simulink model "chap7_8sim"  (Simulink 10.3)
settings: Solver=ode45  StartTime=0.0  StopTime=6  RelTol=1e-3  EnableMultiTasking=on
settings Model: Creator=shipe  LastModifiedBy=shipe
settings SolverCC: AlgebraicLoopSolver=Auto
settings DataIOCC: LimitDataPoints=on  SignalLoggingName=sigsOut
settings OptimizationCC: ExpressionDepthLimit=128  LifeSpan=auto
settings DebuggingCC: SaveWithParameterizedLinksMsg=none  SignalResolutionControl=TryResolveAllWithWarning  MultiTaskDSMMsg=warning  MultiTaskCondExecSysMsg=none  FcnCallInpInsideContextMsg=error  StateNameClashWarn=none  SFUnexpectedBacktrackingDiag=error  SFNoUnconditionalDefaultTransitionDiag=error  SFExecutionAtInitializationDiag=warning  SFMachineParentedDataDiag=error  ArithmeticOperatorsInVariantConditions=error
settings HardwareCC: TargetUnknown=on
settings SFSimCC: SimUseLocalCustomCode=on  CustomCodeUndefinedFunction=FilterOut
settings RTWCC: RTWUseLocalCustomCode=on
settings CodeAppCC: StateflowObjectComments=off
settings GRTTargetCC: TargetLangStandard=C99 (ISO)
settings ConfigComp: CovExternalEMLEnable=on

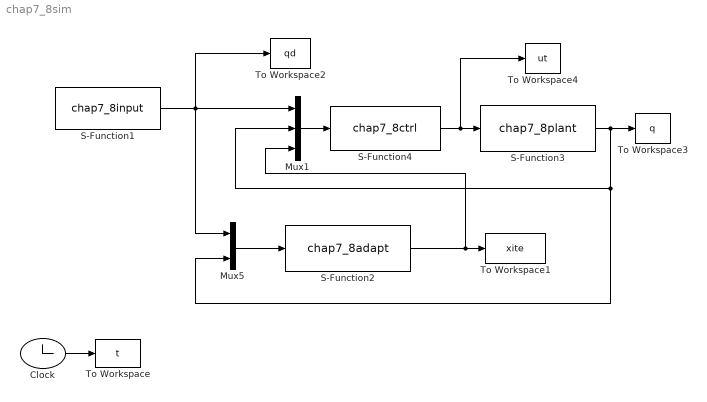
== system chap7_8sim ==
  Clock : Clock
  Mux1 : Mux  Inputs=3
  Mux5 : Mux  Inputs=2
  S-Function1 : S-Function  FunctionName=chap7_8input  SFunctionDeploymentMode=off  EnableBusSupport=off
  S-Function2 : S-Function  FunctionName=chap7_8adapt  SFunctionDeploymentMode=off  EnableBusSupport=off
  S-Function3 : S-Function  FunctionName=chap7_8plant  SFunctionDeploymentMode=off  EnableBusSupport=off
  S-Function4 : S-Function  FunctionName=chap7_8ctrl  SFunctionDeploymentMode=off  EnableBusSupport=off
  To Workspace : ToWorkspace  VariableName=t  SampleTime=-1
  To Workspace1 : ToWorkspace  VariableName=xite  SampleTime=-1
  To Workspace2 : ToWorkspace  VariableName=qd  SampleTime=-1
  To Workspace3 : ToWorkspace  VariableName=q  SampleTime=-1
  To Workspace4 : ToWorkspace  VariableName=ut  SampleTime=-1
  wires:
  S-Function4/1 -> S-Function3/1, To Workspace4/1
  S-Function3/1 -> Mux5/2, Mux1/2, To Workspace3/1
  Mux5/1 -> S-Function2/1
  Mux1/1 -> S-Function4/1
  S-Function1/1 -> Mux1/1, Mux5/1, To Workspace2/1
  S-Function2/1 -> To Workspace1/1, Mux1/3
  Clock/1 -> To Workspace/1
